simulink subsystem "forces"  (R2024b)
settings: Solver=VariableStepAuto  StartTime=0.0  StopTime=10.0  RelTol=1e-3
undefined symbols (not defined in the file): refa, refl
settings Model: Creator=yagiz  LastModifiedBy=yagiz

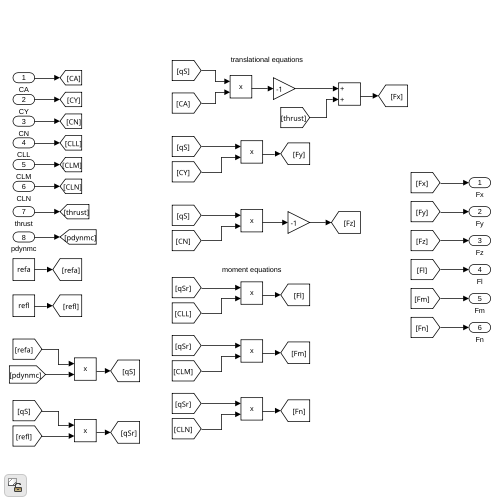
[thumbnail: Simulink's stored preview of the top-level diagram]
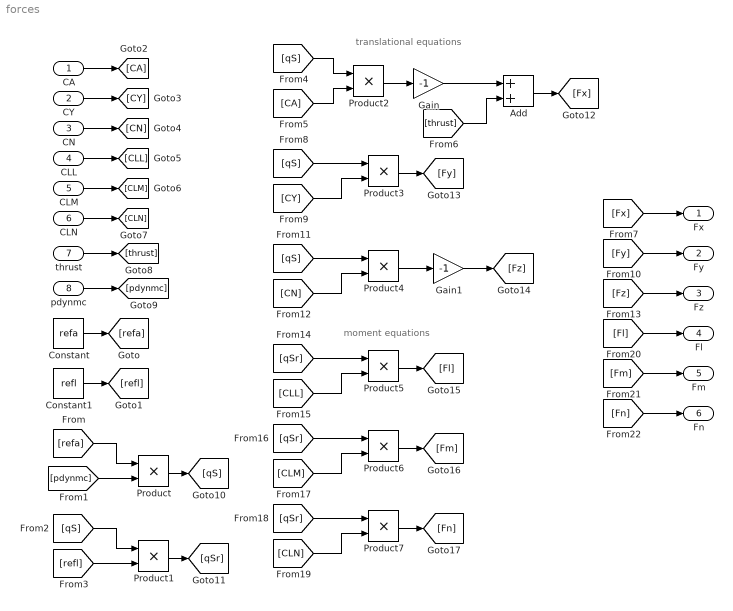
== system forces ==
  note: translational equations
  note: moment equations
  CA : Inport
  CY : Inport  Port=2
  CN : Inport  Port=3
  CLL : Inport  Port=4
  CLM : Inport  Port=5
  CLN : Inport  Port=6
  thrust : Inport  Port=7
  pdynmc : Inport  Port=8
  Add : Sum
  Constant : Constant  Value=refa
  Constant1 : Constant  Value=refl
  Gain : Gain  Gain=-1
  Gain1 : Gain  Gain=-1
  Product{,1..7} (8 alike) : Product
  Fx : Outport
  Fy : Outport  Port=2
  Fz : Outport  Port=3
  Fl : Outport  Port=4
  Fm : Outport  Port=5
  Fn : Outport  Port=6
  wires:
  Constant/1 -> [refa]
  Constant1/1 -> [refl]
  [refa] -> Product/1
  CA/1 -> [CA]
  CY/1 -> [CY]
  CN/1 -> [CN]
  CLL/1 -> [CLL]
  CLM/1 -> [CLM]
  CLN/1 -> [CLN]
  thrust/1 -> [thrust]
  pdynmc/1 -> [pdynmc]
  [pdynmc] -> Product/2
  Product/1 -> [qS]
  [refl] -> Product1/2
  Product1/1 -> [qSr]
  [qS] -> Product1/1
  [qS] -> Product2/1
  [CA] -> Product2/2
  Product2/1 -> Gain/1
  Gain/1 -> Add/1
  [thrust] -> Add/2
  Add/1 -> [Fx]
  [Fx] -> Fx/1
  [qS] -> Product3/1
  [CY] -> Product3/2
  Product3/1 -> [Fy]
  [Fy] -> Fy/1
  Product4/1 -> Gain1/1
  [CN] -> Product4/2
  [qS] -> Product4/1
  Gain1/1 -> [Fz]
  [Fz] -> Fz/1
  Product5/1 -> [Fl]
  [CLL] -> Product5/2
  [qSr] -> Product5/1
  Product6/1 -> [Fm]
  [CLM] -> Product6/2
  [qSr] -> Product6/1
  Product7/1 -> [Fn]
  [CLN] -> Product7/2
  [qSr] -> Product7/1
  [Fl] -> Fl/1
  [Fm] -> Fm/1
  [Fn] -> Fn/1
